simulink model "MechanicalParameterEKF_"  (R2019b)
settings: Solver=VariableStepAuto  StartTime=0.0  StopTime=10.0  RelTol=1e-3
PreLoadFcn:
  | modelDir = fileparts(get_param(bdroot, 'FileName'));
  | addpath(fullfile(modelDir,'../../Parameters'));
  | addpath(fullfile(modelDir,'../../Estimation/MechanicalParameters'));
  | 
  | Parameters_Model
  | Parameters_Simulation
  | Parameters_Estimators
InitFcn:
  | Parameters_Model
  | Parameters_Simulation
  | Parameters_Estimators
undefined symbols (not defined in the file): JKeBTauCekf_P_init, JKeBTauCekf_X_init, Kt, R
settings Model: Creator=Thomas  LastModifiedBy=thomas.jespersen
settings DataIOCC: ReturnWorkspaceOutputs=off
settings DebuggingCC: ArithmeticOperatorsInVariantConditions=warning
settings SFSimCC: SimUseLocalCustomCode=off  CustomCodeUndefinedFunction=UseInterfaceOnly
settings RTWCC: RTWUseLocalCustomCode=off

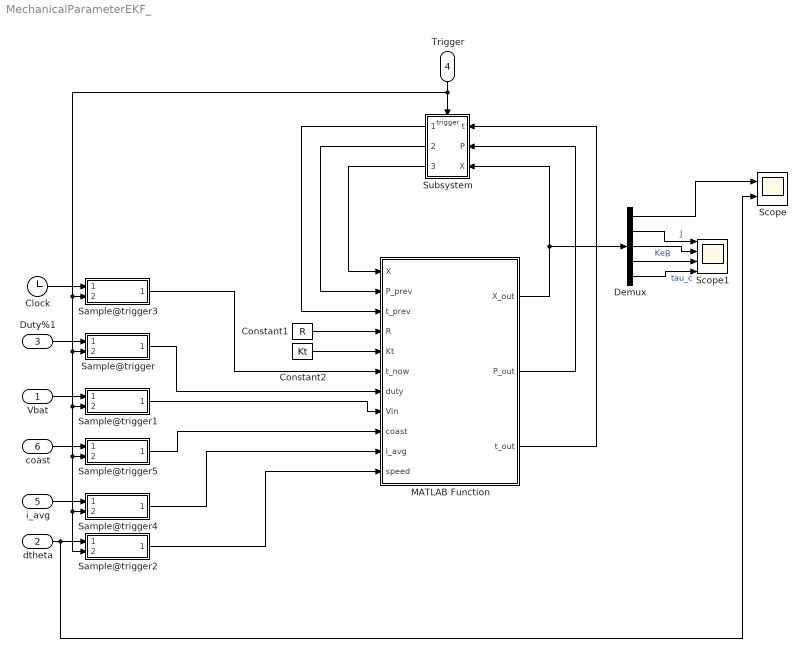
== system MechanicalParameterEKF_ ==
  Vbat : Inport  OutDataTypeStr=double
  dtheta : Inport  Port=2  OutDataTypeStr=double
  Duty%1 : Inport  Port=3  OutDataTypeStr=double
  Trigger : Inport  Port=4  OutDataTypeStr=boolean
  i_avg : Inport  Port=5  OutDataTypeStr=double
  coast : Inport  Port=6  OutDataTypeStr=boolean
  Clock : Clock
  Constant1 : Constant  Value=R
  Constant2 : Constant  Value=Kt
  Demux : Demux  Outputs=5
  MATLAB Function : MATLAB Function  TreatAsAtomicUnit=on
  Sample@trigger : Subsystem
  Sample@trigger1 : Subsystem
  Sample@trigger2 : Subsystem
  Sample@trigger3 : Subsystem
  Sample@trigger4 : Subsystem
  Sample@trigger5 : Subsystem
  Scope : Scope  NumInputPorts=2
  Scope1 : Scope  NumInputPorts=4
  Subsystem : Subsystem
  wires:
  MATLAB Function/1(X_out) -> Demux/1, Subsystem/3(X)
  MATLAB Function/2(P_out) -> Subsystem/2(P)
  Subsystem/2(P_prev) -> MATLAB Function/2(P_prev)
  Subsystem/3(X_prev) -> MATLAB Function/1(X)
  Constant1/1 -> MATLAB Function/4(R)
  Constant2/1 -> MATLAB Function/5(Kt)
  Duty%1/1 -> Sample@trigger/1(Signal)
  Trigger/1 -> Sample@trigger3/2(Trigger), Sample@trigger1/2(Trigger), Sample@trigger5/2(Trigger), Sample@trigger4/2(Trigger), Sample@trigger2/2(Trigger), Sample@trigger/2(Trigger), Subsystem/Trigger
  Vbat/1 -> Sample@trigger1/1(Signal)
  dtheta/1 -> Scope/2, Sample@trigger2/1(Signal)
  Sample@trigger/1(Sample) -> MATLAB Function/7(duty)
  Sample@trigger1/1(Sample) -> MATLAB Function/8(Vin)
  Sample@trigger2/1(Sample) -> MATLAB Function/11(speed)
  Subsystem/1(t_prev) -> MATLAB Function/3(t_prev)
  MATLAB Function/3(t_out) -> Subsystem/1(t)
  Clock/1 -> Sample@trigger3/1(Signal)
  Sample@trigger3/1(Sample) -> MATLAB Function/6(t_now)
  Sample@trigger4/1(Sample) -> MATLAB Function/10(i_avg)
  i_avg/1 -> Sample@trigger4/1(Signal)
  Sample@trigger5/1(Sample) -> MATLAB Function/9(coast)
  coast/1 -> Sample@trigger5/1(Signal)
  Demux/1 -> Scope/1
  Demux/2 -> Scope1/1  "J"
  Demux/3 -> Scope1/2  "Ke"
  Demux/4 -> Scope1/3  "B"
  Demux/5 -> Scope1/4  "tau_c"

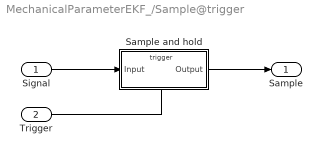
== system MechanicalParameterEKF_/Sample@trigger ==
  Signal : Inport
  Trigger : Inport  Port=2
  Sample and hold : Subsystem
  Sample : Outport  VectorParamsAs1DForOutWhenUnconnected=off
  wires:
  Signal/1 -> Sample and hold/1(Input)
  Sample and hold/1(Output) -> Sample/1
  Trigger/1 -> Sample and hold/Trigger

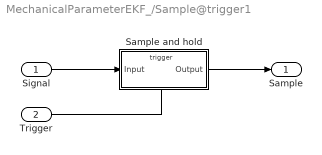
== system MechanicalParameterEKF_/Sample@trigger1 ==
  Signal : Inport
  Trigger : Inport  Port=2
  Sample and hold : Subsystem
  Sample : Outport  VectorParamsAs1DForOutWhenUnconnected=off
  wires:
  Signal/1 -> Sample and hold/1(Input)
  Sample and hold/1(Output) -> Sample/1
  Trigger/1 -> Sample and hold/Trigger

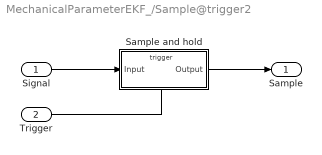
== system MechanicalParameterEKF_/Sample@trigger2 ==
  Signal : Inport
  Trigger : Inport  Port=2
  Sample and hold : Subsystem
  Sample : Outport  VectorParamsAs1DForOutWhenUnconnected=off
  wires:
  Signal/1 -> Sample and hold/1(Input)
  Sample and hold/1(Output) -> Sample/1
  Trigger/1 -> Sample and hold/Trigger

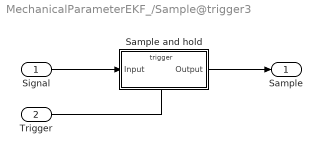
== system MechanicalParameterEKF_/Sample@trigger3 ==
  Signal : Inport
  Trigger : Inport  Port=2
  Sample and hold : Subsystem
  Sample : Outport  VectorParamsAs1DForOutWhenUnconnected=off
  wires:
  Signal/1 -> Sample and hold/1(Input)
  Sample and hold/1(Output) -> Sample/1
  Trigger/1 -> Sample and hold/Trigger

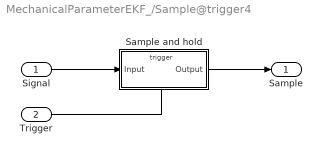
== system MechanicalParameterEKF_/Sample@trigger4 ==
  Signal : Inport
  Trigger : Inport  Port=2
  Sample and hold : Subsystem
  Sample : Outport  VectorParamsAs1DForOutWhenUnconnected=off
  wires:
  Signal/1 -> Sample and hold/1(Input)
  Sample and hold/1(Output) -> Sample/1
  Trigger/1 -> Sample and hold/Trigger

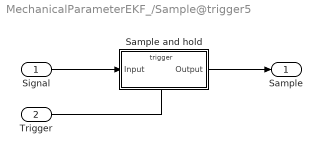
== system MechanicalParameterEKF_/Sample@trigger5 ==
  Signal : Inport
  Trigger : Inport  Port=2
  Sample and hold : Subsystem
  Sample : Outport  VectorParamsAs1DForOutWhenUnconnected=off
  wires:
  Signal/1 -> Sample and hold/1(Input)
  Sample and hold/1(Output) -> Sample/1
  Trigger/1 -> Sample and hold/Trigger

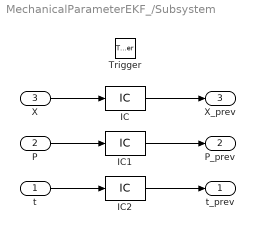
== system MechanicalParameterEKF_/Subsystem ==
  t : Inport  LatchByDelayingOutsideSignal=on
  P : Inport  Port=2  LatchByDelayingOutsideSignal=on
  X : Inport  Port=3  LatchByDelayingOutsideSignal=on
  Trigger : TriggerPort  VariantControl=Variant  PortDimensions=1
  IC : InitialCondition  Value=JKeBTauCekf_X_init
  IC1 : InitialCondition  Value=JKeBTauCekf_P_init
  IC2 : InitialCondition  Value=0
  t_prev : Outport  VectorParamsAs1DForOutWhenUnconnected=off
  P_prev : Outport  Port=2  VectorParamsAs1DForOutWhenUnconnected=off
  X_prev : Outport  Port=3  VectorParamsAs1DForOutWhenUnconnected=off
  wires:
  X/1 -> IC/1
  P/1 -> IC1/1
  IC/1 -> X_prev/1
  IC1/1 -> P_prev/1
  IC2/1 -> t_prev/1
  t/1 -> IC2/1

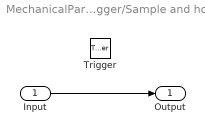
== system MechanicalParameterEKF_/Sample@trigger/Sample and hold ==
  Input : Inport
  Trigger : TriggerPort  VariantControl=Variant  PortDimensions=1
  Output : Outport  VectorParamsAs1DForOutWhenUnconnected=off
  wires:
  Input/1 -> Output/1

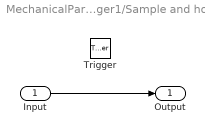
== system MechanicalParameterEKF_/Sample@trigger1/Sample and hold ==
  Input : Inport
  Trigger : TriggerPort  VariantControl=Variant  PortDimensions=1
  Output : Outport  VectorParamsAs1DForOutWhenUnconnected=off
  wires:
  Input/1 -> Output/1

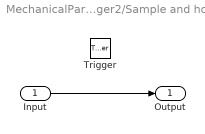
== system MechanicalParameterEKF_/Sample@trigger2/Sample and hold ==
  Input : Inport
  Trigger : TriggerPort  VariantControl=Variant  PortDimensions=1
  Output : Outport  VectorParamsAs1DForOutWhenUnconnected=off
  wires:
  Input/1 -> Output/1

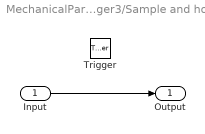
== system MechanicalParameterEKF_/Sample@trigger3/Sample and hold ==
  Input : Inport
  Trigger : TriggerPort  VariantControl=Variant  PortDimensions=1
  Output : Outport  VectorParamsAs1DForOutWhenUnconnected=off
  wires:
  Input/1 -> Output/1

== system MechanicalParameterEKF_/Sample@trigger4/Sample and hold ==
  Input : Inport
  Trigger : TriggerPort  VariantControl=Variant  PortDimensions=1
  Output : Outport  VectorParamsAs1DForOutWhenUnconnected=off
  wires:
  Input/1 -> Output/1

== system MechanicalParameterEKF_/Sample@trigger5/Sample and hold ==
  Input : Inport
  Trigger : TriggerPort  VariantControl=Variant  PortDimensions=1
  Output : Outport  VectorParamsAs1DForOutWhenUnconnected=off
  wires:
  Input/1 -> Output/1

== matlab function MechanicalParameterEKF_/MATLAB Function ==
  data: X input; X_out output; P_prev input; t_prev input; R input; Kt input; t_now input; duty input; Vin input; coast input; i_avg input; speed input; P_out output; t_out output
function [X_out, P_out, t_out] = MechanicalParameterEKF_(X, P_prev, t_prev, ...
    R, Kt, ... % constants/parameters
    t_now, duty, Vin, coast, ... % inputs (u)
    i_avg, speed)  % measurements (z)

    [X_out, P_out, t_out] = MechanicalParameterEKF(X, P_prev, t_prev, ...
        R, Kt, ... % constants/parameters
        t_now, duty, Vin, coast, ... % inputs (u)
        i_avg, speed);  % measurements (z)

end
